simulink model "diagrama_simulink"  (R2015a)
settings: Solver=ode45  StartTime=0.0  StopTime=t_train(end)  RelTol=1e-3
values from neighbouring files (symbols this model uses):
  b = 0.1    [codigo.m]
  J = 1    [codigo.m]
  K = 1    [codigo.m]
  kpwm = 30    [codigo.m]
  La = 369.5e-3    (= 0.3695)    [codigo.m]
  Ra = 38.8755    [codigo.m]
settings Model: Creator=FURRUSCAR  LastModifiedBy=FURRUSCAR

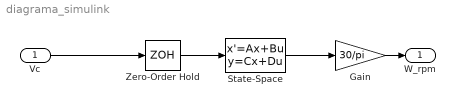
== system diagrama_simulink ==
  Vc : Inport
  Gain : Gain  Gain=30/pi
  State-Space : StateSpace  A=[-Ra/La -K/La;K/J -b/J]  B=[kpwm/La;0]  C=[0 1]  D=0  X0=0
  Zero-Order Hold : ZeroOrderHold  SampleTime=0.1
  "W_rpm " : Outport
  wires:
  Zero-Order Hold/1 -> State-Space/1
  ? -> ?
  Vc/1 -> Zero-Order Hold/1
  State-Space/1 -> Gain/1
  Gain/1 -> "W_rpm "/1
